simulink model "PV_Geno_VSC_GFL_634"  (R2024b)
settings: Solver=ode5  StartTime=0.0  StopTime=5  MaxStep=1e-4  RelTol=1e-6  AbsTol=1e-8
values from neighbouring files (symbols this model uses):
  a = 1.3    [init_para_with_symmtrc_loads.m]
  amp_ptb = amp_rel*Vp    [a01_scan_VSC_13_feeder.m]
  Cdc = 278e-3    (= 0.278)    [init_para_with_symmtrc_loads.m]
  fg = 60    [a01_scan_VSC_13_feeder.m]    (also in init_para_with_symmtrc_loads.m)
  Gn = 1000    [init_para_with_symmtrc_loads.m]
  Ipv_n = Isc_n*(Rp+Rs)/Rp    (= 8.21426513558)    [init_para_with_symmtrc_loads.m]
  Isc_n = 8.21    [init_para_with_symmtrc_loads.m]
  k = 1.3806503e-23    [init_para_with_symmtrc_loads.m]    (also in ypm_plot_compare_ana_meas.m = 2)
  KI = 0.0032    [init_para_with_symmtrc_loads.m]
  Ki_C = Rc/tau_C    (= 0.768)    [init_para_with_symmtrc_loads.m]
  Ki_DC = omega_DC^2*Cdc    [init_para_with_symmtrc_loads.m]
  Ki_P = 1/(Ki_pq*tau_P)    [init_para_with_symmtrc_loads.m]
  Ki_PLL = Kp_PLL/tau_PLL    [init_para_with_symmtrc_loads.m]
  Kp_C = Lc/tau_C    (= 0.020372)    [init_para_with_symmtrc_loads.m]
  Kp_DC = 2*xi_DC*omega_DC*Cdc    [init_para_with_symmtrc_loads.m]
  Kp_P = tau_C/(Ki_pq*tau_P)    [init_para_with_symmtrc_loads.m]
  Kp_PLL = xi_PLL*2*omega_PLL/Vp    [init_para_with_symmtrc_loads.m]
  KV = -0.123    [init_para_with_symmtrc_loads.m]
  KVmp = Vmp_n/Voc_n    (= 0.799392097264)    [init_para_with_symmtrc_loads.m]
  Lc = 20.372e-6    (= 2.0372e-05)    [init_para_with_symmtrc_loads.m]
  Np = 345    [init_para_with_symmtrc_loads.m]
  Ns = 45    [init_para_with_symmtrc_loads.m]
  Ns_cell = 54    [init_para_with_symmtrc_loads.m]
  phi_ptb = phi_ptb_vec(run)    [a01_scan_VSC_13_feeder.m]
  phs0 = mod(-w_ptb*t_start, 2*pi)    [a01_scan_VSC_13_feeder.m]
  psi_0 = 0    [a01_scan_VSC_13_feeder.m]
  q = 1.6021764e-19    [init_para_with_symmtrc_loads.m]
  Rc = 0.768e-3    (= 0.000768)    [init_para_with_symmtrc_loads.m]
  Rp = 425.405    [init_para_with_symmtrc_loads.m]
  Rs = 0.221    [init_para_with_symmtrc_loads.m]
  S_base_all = 1    [init_para_with_symmtrc_loads.m]
  t_start = t_settle    (= 0.5)    [a01_scan_VSC_13_feeder.m]
  Tn = 25    [init_para_with_symmtrc_loads.m]
  Ts = T_ctrl/n_ctrl    [a01_scan_VSC_13_feeder.m]    (also in init_para_with_symmtrc_loads.m = 5e-05)
  Vdc = 1200    [init_para_with_symmtrc_loads.m]
  Voc_n = 32.9    [init_para_with_symmtrc_loads.m]
  Vp = sqrt(2)*480/sqrt(3)    [a01_scan_VSC_13_feeder.m]    (also in init_para_with_symmtrc_loads.m = Ug*sqrt(2)/sqrt(3))
  w_ptb = 2*pi*fp    [a01_scan_VSC_13_feeder.m]
undefined symbols (not defined in the file or in its folder): Amp_ptb_A, Amp_ptb_B, Amp_ptb_C, DiscIntNeverNeededParam, frq_ptb_A, frq_ptb_B, frq_ptb_C, j, para_PVgeno, phs_ptb_A, phs_ptb_B, phs_ptb_C
libraries: spsControlledVoltageSourceLib x6, slpidlib x5, spsSeriesRLCBranchLib x4, spsPower3phInstantaneousLib x2, spsabctoAlphaBetaZeroLib x2, spsCurrentMeasurementLib x2, spsControlledCurrentSourceLib x2, spsGroundLib x1, spsVoltageMeasurementLib x1, spsThreePhaseVIMeasurementLib x1, spsThreePhaseParallelRLCLoadLib x1, spsThreePhaseSourceLib x1
(part 1 of 2)
settings Model: Creator=clubbert  LastModifiedBy=clubbert
settings DataIOCC: Decimation=D_log  SaveOutput=off  SaveState=on  DSMLogging=off

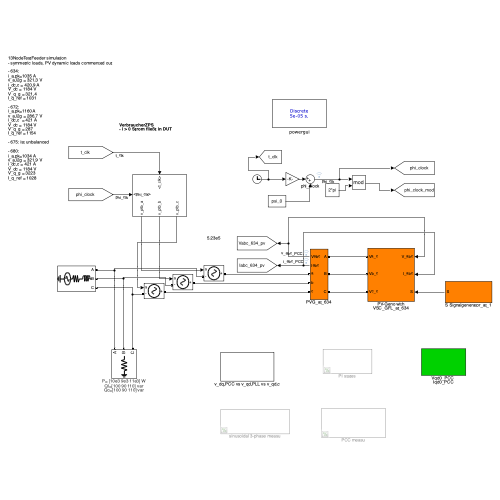
[thumbnail: Simulink's stored preview of the top-level diagram]
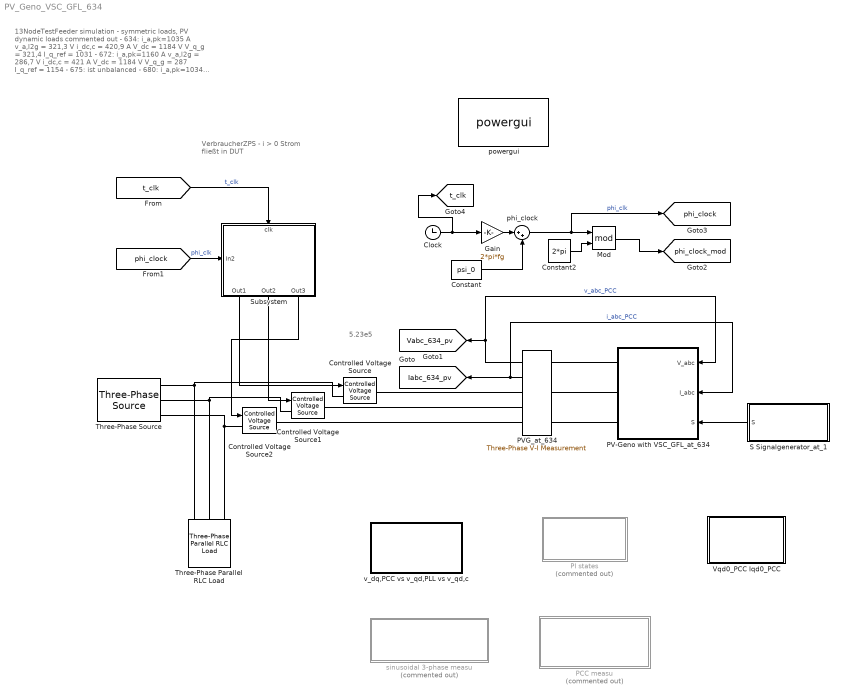
== system PV_Geno_VSC_GFL_634 ==
  note: VerbraucherZPS
      | - i > 0 Strom fließt in DUT
  note: 13NodeTestFeeder simulation
      | - symmetric loads, PV dynamic loads commented out
      |
      | - 634:
      | i_a,pk=1035 A
      | v_a,l2g = 321,3 V
      | i_dc,c = 420,9 A
      | V_dc = 1184 V
      | V_q_g = 321,4
      | I_q_ref = 1031
      |
      | - 672:
      | i_a,pk=1160 A
      | v_a,l2g = 286,7 V
      | i_dc,c  = 421 A
      | V_dc = 1184 V
      | V_q_g = 287
      | I_q_ref = 1154
      |
      | - 675: ist unbalanced
      |
      | - 680:
      | i_a,pk=1034 A
      | v_a,l2g = 321,9 V
      | i_dc,c = 421 A
      | V_dc = 1184 V
      | V_q_g = 3223
      | I_q_ref = 1028
  note: 5.23e5
  Clock : Clock
  Constant : Constant  Value=psi_0
  Constant2 : Constant  Value=2*pi
  Controlled Voltage Source : spsControlledVoltageSourceLib/Controlled Voltage Source  Initialize=on  Source_Type=AC  Amplitude=0  Phase=0  Frequency=0  Measurements=None
  Controlled Voltage Source1 : spsControlledVoltageSourceLib/Controlled Voltage Source  Initialize=on  Source_Type=AC  Amplitude=0  Phase=0  Frequency=0  Measurements=None
  Controlled Voltage Source2 : spsControlledVoltageSourceLib/Controlled Voltage Source  Initialize=on  Source_Type=AC  Amplitude=0  Phase=0  Frequency=0  Measurements=None
  Gain : Gain  Gain=2*pi*fg
  Mod : Math  Operator=mod
  PCC measu : Subsystem  Commented=on
  PI states : Subsystem  Commented=on
  "PV-Geno with VSC_GFL_at_634     " : Subsystem
      settings: PortSchema="{\"entries\":[{\"content\":{\"sides\":[{\"content\":{\"connectorIds\":[\"LConn1\",\"LConn2\",\"LConn3\"]},\"type\":\"ConnectorPlacement.EquallySpacedRectSide\",\"uuid\":\"92a05cf9-a19b-475d-bffb-9406018f82f4\"},{\"content\":{\"connectorIds\":[\"In1\",\"In2\",\"In3\"],\"side\":\"RIGHT\"},\"type\":\"ConnectorPlacement.EquallySpacedRectSide\",\"uuid\":\"83076eb6-0a86-49d7-8932-035501cdc6f6\"},{\"content\":{\"side\":\"TOP\"},\"type\":\"ConnectorPlacement.EquallySpacedRectSide\",\"uuid\":\"ba2310df-ee07-4a5c-88ff-ef0f81658322\"}]},\"type\":\"ConnectorPlacement.EquallySpacedConnector\",\"uuid\":\"9e64c472-0dae-4bb4-8eb3-3329c328d412\"}],\"packageUris\":[\"http://schema.mathworks.com/mf0/Connector/R2020b\"],\"version\":\"1.0\"}"
  PVG_at_634 : spsThreePhaseVIMeasurementLib/Three-Phase V-I Measurement  VoltageMeasurement=phase-to-ground  SetLabelV=off  LabelV=V_abc_PCC_634_pv  Vpu=off  VpuLL=off  CurrentMeasurement=yes  SetLabelI=off  LabelI=I_abc_PCC_634_pv  Ipu=off  Pbase=100e6  Vbase=4160  OutputType=Complex  PhasorSimulation=off  PSBequivalent=0
  S Signalgenerator_at_1 : Subsystem
  Subsystem : Subsystem
      settings: PortSchema="{\"entries\":[{\"content\":{\"sides\":[{\"content\":{\"connectorIds\":[\"In1\"]},\"type\":\"ConnectorPlacement.EquallySpacedRectSide\",\"uuid\":\"f4884b02-4acb-4d3a-a4cd-33952d0bc0e4\"},{\"content\":{\"connectorIds\":[\"Out1\",\"Out2\",\"Out3\"],\"side\":\"RIGHT\"},\"type\":\"ConnectorPlacement.EquallySpacedRectSide\",\"uuid\":\"6584eb96-7add-474a-938e-a48a378b8460\"},{\"content\":{\"connectorIds\":[\"In2\"],\"side\":\"TOP\"},\"type\":\"ConnectorPlacement.EquallySpacedRectSide\",\"uuid\":\"b17781d8-b149-4887-b17a-64ae556a6560\"}]},\"type\":\"ConnectorPlacement.EquallySpacedConnector\",\"uuid\":\"0fcb0f1f-785d-43c8-8af7-8220763653f1\"}],\"packageUris\":[\"http://schema.mathworks.com/mf0/Connector/R2020b\"],\"version\":\"1.0\"}"
  Three-Phase Parallel RLC Load : spsThreePhaseParallelRLCLoadLib/Three-Phase Parallel RLC Load  LConnTagsString=A|B|C  Configuration=Y (grounded)  NominalVoltage=480  Vabc=[1e3 1e3 1e3]  Vabcp=[1e3 1e3 1e3]  NominalFrequency=60  UnbalancedPower=off  ActivePower=4.969e+05  InductivePower=0  CapacitivePower=0  Pabc=[10e3 9e3 11e3]  QLabc=[100 90 110]  QCabc=[100 90 110]  Pabcp=[10e3 9e3 11e3]  QLabcp=[100 90 110]  QCabcp=[100 90 110]  Measurements=None  LoadType=constant Z
      settings: AttributesFormatString=|
      | P= %<Pabc> W
      | Ql=%<QLabc> var
      | Qc=%<QCabc> var
  Three-Phase Source : spsThreePhaseSourceLib/Three-Phase Source  InternalConnection=Yg  VoltagePhases=off  Voltage=480  PhaseAngle=0  Voltage_phases=[25e3 25e3 25e3]/sqrt(3)  PhaseAngles_phases=[0 -120 +120]  Frequency=60  NonIdealSource=on  SpecifyImpedance=on  Resistance=0.8929  Inductance=16.58e-3  ShortCircuitLevel=100e6  BaseVoltage=480  XRratio=7  BusType=swing  Pref=10e3  Qref=0  Prefabc=[10e3, 10e3, 10e3]  Qrefabc=[0, 0, 0]  Qmin=-inf  Qmax=inf
  Vqd0_PCC Iqd0_PCC : Subsystem
  phi_clock : Sum  Inputs=|++
  powergui : sps_lib/powergui  Priority=1  SimulationMode=Discrete  SampleTime=Ts  frequency=60  Iterations=50  frequencyindice=0  Pbase=100e3  ErrMax=0.0001  UnitsV=kV  UnitsW=kW  buscounter=0  FunctionMessages=off  echomessages=off  EnableUseOfTLC=off  CurrentSourceSwitches=off  DisableSnubberDevices=off  DisableRonSwitches=off  DisableVfSwitches=off  DisplayEquations=off  AutomaticDiscreteSolvers=off  SolverType=Tustin/Backward Euler (TBE)  Interpol=off  ExternalGateDelay=off  methode=off  Ts=0  x0status=blocks  SPID=off  SwTol=0  HookPort=off  NonlinearTolerance=1e-4  nMaxIteration=100  ContinueOnMaxIteration=off  RestoreLinks=warning  ResistiveCurrentMeasurement=off  Frange=[0:2:500]  Ylog=off  Xlog=on  ShowGrid=off  save=off  variable=ZData  structure=0  ZoomFFT=on  StartTime=0.0  cycles=1  DisplayStyle=1  fundamental=60  FreqAxis=off  MaxFrequency=1000  frequencyindicesteady=1  RmsSteady=1  display=off
  sinusoidal 3-phase measu : Subsystem  Commented=on
  v_dq,PCC vs v_qd,PLL vs v_qd,c : Subsystem
  tag scope: Iabc_634_pv=global, Vabc_634_pv=global, phi_clock=global, phi_clock_mod=global, t_clk=global
  wires:
  S Signalgenerator_at_1/1(S) -> "PV-Geno with VSC_GFL_at_634     "/3(S)
  PVG_at_634/1 -> "PV-Geno with VSC_GFL_at_634     "/1(V_abc), [Vabc_634_pv]  "v_abc_PCC"
  PVG_at_634/2 -> [Iabc_634_pv], "PV-Geno with VSC_GFL_at_634     "/2(I_abc)  "i_abc_PCC"
  Clock/1 -> [t_clk], Gain/1
  Gain/1 -> phi_clock/1
  phi_clock/1 -> Mod/1, [phi_clock]  "phi_clk"
  Constant/1 -> phi_clock/2
  Constant2/1 -> Mod/2
  Mod/1 -> [phi_clock_mod]
  Subsystem/1(Out1) -> Controlled Voltage Source/1
  Subsystem/2(Out2) -> Controlled Voltage Source1/1
  Subsystem/3(Out3) -> Controlled Voltage Source2/1
  [t_clk] -> Subsystem/1(clk)  "t_clk"
  [phi_clock] -> Subsystem/2(In2)  "phi_clk"
  connections:
  PVG_at_634/RConn3 -- Controlled Voltage Source2/RConn1
  "PV-Geno with VSC_GFL_at_634     "/LConn3 -- PVG_at_634/LConn3
  PVG_at_634/RConn2 -- Controlled Voltage Source1/RConn1
  PVG_at_634/RConn1 -- Controlled Voltage Source/RConn1
  "PV-Geno with VSC_GFL_at_634     "/LConn2 -- PVG_at_634/LConn2
  "PV-Geno with VSC_GFL_at_634     "/LConn1 -- PVG_at_634/LConn1
  Three-Phase Source/RConn1 -- Three-Phase Parallel RLC Load/LConn1 -- Controlled Voltage Source/LConn1
  Three-Phase Source/RConn2 -- Three-Phase Parallel RLC Load/LConn2 -- Controlled Voltage Source1/LConn1
  Three-Phase Source/RConn3 -- Three-Phase Parallel RLC Load/LConn3 -- Controlled Voltage Source2/LConn1

== system PV_Geno_VSC_GFL_634/PCC measu ==
  PQ_4 : Subsystem
  Scope1 : Scope
  Scope2 : Scope  NumInputPorts=2
  wires:
  PQ_4/1(PQ) -> Scope1/1  "PQ_at_634"
  [Iabc_634_pv] -> PQ_4/2(I), Scope2/2  "Iabc"
  [Vabc_634_pv] -> PQ_4/1(U), Scope2/1  "Vabc"

== system PV_Geno_VSC_GFL_634/PI states ==
  Constant : Constant  Value=2*pi*fg*0
  Scope3 : Scope  NumInputPorts=5
  Sum : Sum  Inputs=|++
  wires:
  [y_PI_PLL] -> Sum/2  "y_PI_PLL"
  [y_PI_q_CC] -> Scope3/4  "y_PI_q_CC"
  [y_PI_q_CC] -> Scope3/5  "y_PI_q_CC"
  [y_PI_DC] -> Scope3/2  "y_PI_DC"
  [y_PI_QC] -> Scope3/3  "y_PI_QC"
  Constant/1 -> Sum/1
  Sum/1 -> Scope3/1

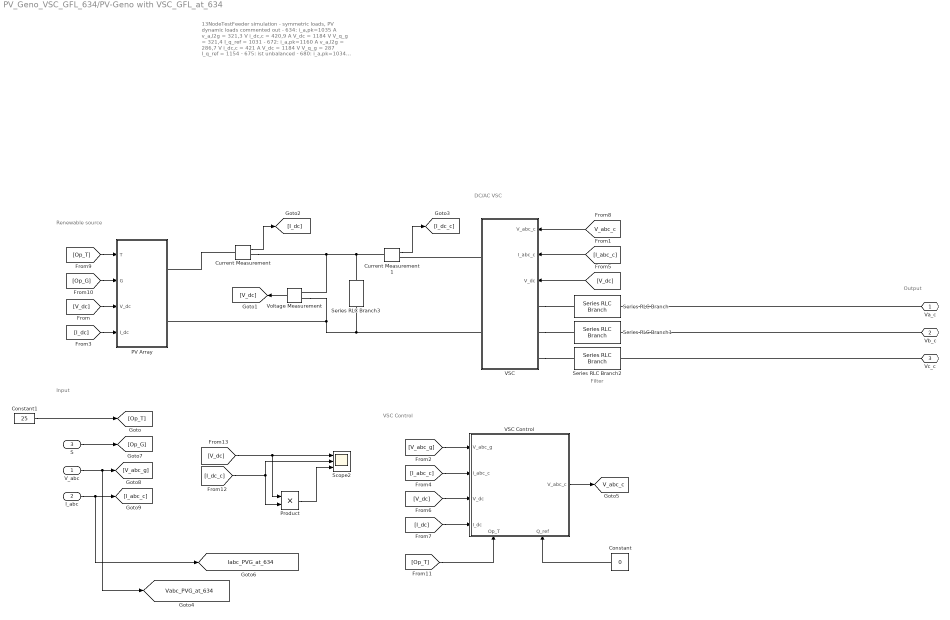
== system PV_Geno_VSC_GFL_634/PV-Geno with VSC_GFL_at_634      ==
  note: 13NodeTestFeeder simulation
      | - symmetric loads, PV dynamic loads commented out
      |
      | - 634:
      | i_a,pk=1035 A
      | v_a,l2g = 321,3 V
      | i_dc,c = 420,9 A
      | V_dc = 1184 V
      | V_q_g = 321,4
      | I_q_ref = 1031
      |
      | - 672:
      | i_a,pk=1160 A
      | v_a,l2g = 286,7 V
      | i_dc,c  = 421 A
      | V_dc = 1184 V
      | V_q_g = 287
      | I_q_ref = 1154
      |
      | - 675: ist unbalanced
      |
      | - 680:
      | i_a,pk=1034 A
      | v_a,l2g = 321,9 V
      | i_dc,c = 421 A
      | V_dc = 1184 V
      | V_q_g = 3223
      | I_q_ref = 1028
  note: Output
  note: Input
  note: Filter
  note: Renewable source
  note: VSC Control
  note: DC/AC VSC
  V_abc : Inport
  I_abc : Inport  Port=2
  S : Inport  Port=3
  Constant : Constant  Value=0
  Constant1 : Constant  Value=25
  Current Measurement : spsCurrentMeasurementLib/Current Measurement  PhasorSimulation=off  OutputType=Complex  PSBequivalent=0
  Current Measurement1 : spsCurrentMeasurementLib/Current Measurement  PhasorSimulation=off  OutputType=Complex  PSBequivalent=0
  PV Array : Subsystem
  Product : Product
  Scope2 : Scope  NumInputPorts=3
  Series RLC Branch : spsSeriesRLCBranchLib/Series RLC Branch  LConnTagsString=__new0  RConnTagsString=__new0  BranchType=RL  Resistance=Rc  Inductance=Lc  SetiL0=off  InitialCurrent=0  Capacitance=1e-6  Setx0=off  InitialVoltage=0  Measurements=None
  Series RLC Branch1 : spsSeriesRLCBranchLib/Series RLC Branch  LConnTagsString=__new0  RConnTagsString=__new0  BranchType=RL  Resistance=Rc  Inductance=Lc  SetiL0=off  InitialCurrent=0  Capacitance=1e-6  Setx0=off  InitialVoltage=0  Measurements=None
  Series RLC Branch2 : spsSeriesRLCBranchLib/Series RLC Branch  LConnTagsString=__new0  RConnTagsString=__new0  BranchType=RL  Resistance=Rc  Inductance=Lc  SetiL0=off  InitialCurrent=0  Capacitance=1e-6  Setx0=off  InitialVoltage=0  Measurements=None
  Series RLC Branch3 : spsSeriesRLCBranchLib/Series RLC Branch  LConnTagsString=__new0  RConnTagsString=__new0  BranchType=C  Resistance=0.3  Inductance=1e-3  SetiL0=off  InitialCurrent=0  Capacitance=Cdc  Setx0=on  InitialVoltage=Vdc  Measurements=None
  VSC : Subsystem
  VSC Control : Subsystem
      settings: PortSchema="{\"entries\":[{\"content\":{\"sides\":[{\"content\":{\"connectorIds\":[\"In1\",\"In2\",\"In3\",\"In4\"]},\"type\":\"ConnectorPlacement.EquallySpacedRectSide\",\"uuid\":\"1f0c866f-1355-4493-8a8b-fecd52da2e06\"},{\"content\":{\"connectorIds\":[\"Out1\"],\"side\":\"RIGHT\"},\"type\":\"ConnectorPlacement.EquallySpacedRectSide\",\"uuid\":\"e0482316-46fe-491c-835b-46d73fa6817a\"},{\"content\":{\"side\":\"TOP\"},\"type\":\"ConnectorPlacement.EquallySpacedRectSide\",\"uuid\":\"b85aba4d-c629-42a9-b30e-3179992b26cb\"},{\"content\":{\"connectorIds\":[\"In5\",\"In6\"],\"side\":\"BOTTOM\"},\"type\":\"ConnectorPlacement.EquallySpacedRectSide\",\"uuid\":\"2c79aeba-fb98-4b17-8331-d72a75796cf8\"}]},\"type\":\"ConnectorPlacement.EquallySpacedConnector\",\"uuid\":\"5586ce08-6872-4275-b1b0-323c6fc0897a\"}],\"packageUris\":[\"http://schema.mathworks.com/mf0/Connector/R2020b\"],\"version\":\"1.0\"}"
  Voltage Measurement : spsVoltageMeasurementLib/Voltage Measurement  PhasorSimulation=off  OutputType=Complex  PSBequivalent=0
  Va_c : PMIOPort  Side=Left
  Vb_c : PMIOPort  Port=2  Side=Left
  Vc_c : PMIOPort  Port=3  Side=Left
  tag scope: Iabc_PVG_at_634=global, V_abc_c=global, Vabc_PVG_at_634=global
  wires:
  [V_abc_c] -> VSC/1(V_abc_c)
  Constant/1 -> VSC Control/6(Q_ref)
  Current Measurement1/1 -> [I_dc_c]
  [V_dc] -> Scope2/1, Product/1
  [I_dc_c] -> Scope2/2, Product/2
  [I_dc] -> VSC Control/4(I_dc)
  Voltage Measurement/1 -> [V_dc]
  [V_abc_g] -> VSC Control/1(V_abc_g)
  VSC Control/1(V_abc_c) -> [V_abc_c]
  [V_dc] -> PV Array/3(V_dc)
  Current Measurement/1 -> [I_dc]
  Product/1 -> Scope2/3
  [Op_T] -> VSC Control/5(Op_T)
  [V_dc] -> VSC/3(V_dc)
  V_abc/1 -> [Vabc_PVG_at_634], [V_abc_g]
  [Op_T] -> PV Array/1(T)
  [V_dc] -> VSC Control/3(V_dc)
  [Op_G] -> PV Array/2(G)
  [I_abc_c] -> VSC Control/2(I_abc_c)
  [I_abc_c] -> VSC/2(I_abc_c)
  [I_dc] -> PV Array/4(I_dc)
  S/1 -> [Op_G]
  Constant1/1 -> [Op_T]
  I_abc/1 -> [Iabc_PVG_at_634], [I_abc_c]
  connections:
  VSC/LConn2 -- Series RLC Branch1/RConn1
  Series RLC Branch3/RConn1 -- Voltage Measurement/LConn2 -- PV Array/RConn2 -- VSC/RConn2
  Current Measurement1/LConn1 -- Series RLC Branch3/LConn1 -- Current Measurement/RConn1 -- Voltage Measurement/LConn1
  Current Measurement/LConn1 -- PV Array/RConn1
  VSC/LConn1 -- Series RLC Branch/RConn1
  VSC/LConn3 -- Series RLC Branch2/RConn1
  Va_c/RConn1 -- Series RLC Branch/LConn1
  VSC/RConn1 -- Current Measurement1/RConn1
  Vc_c/RConn1 -- Series RLC Branch2/LConn1
  Vb_c/RConn1 -- Series RLC Branch1/LConn1

== system PV_Geno_VSC_GFL_634/S Signalgenerator_at_1 ==
  Constant : Constant  Value=para_PVgeno.S_ini1
  Product : Product  Commented=on
  Signal Generator : SignalGenerator  Commented=on  Amplitude=50  Frequency=0.25
  Step : Step  Commented=on  Time=para_PVgeno.t_step  After=para_PVgeno.S_step  SampleTime=0
  Step1 : Step  Commented=on  Time=para_PVgeno.t_step11  After=para_PVgeno.S_step11  SampleTime=0
  Step2 : Step  Time=para_PVgeno.t_step12  After=para_PVgeno.S_step12  SampleTime=0
  Sum : Sum  Inputs=|++++
  S : Outport
  wires:
  Sum/1 -> S/1
  Constant/1 -> Sum/1
  Step2/1 -> Sum/3
  Step1/1 -> Product/1
  Signal Generator/1 -> Product/2
  Product/1 -> Sum/2
  Step/1 -> Sum/4

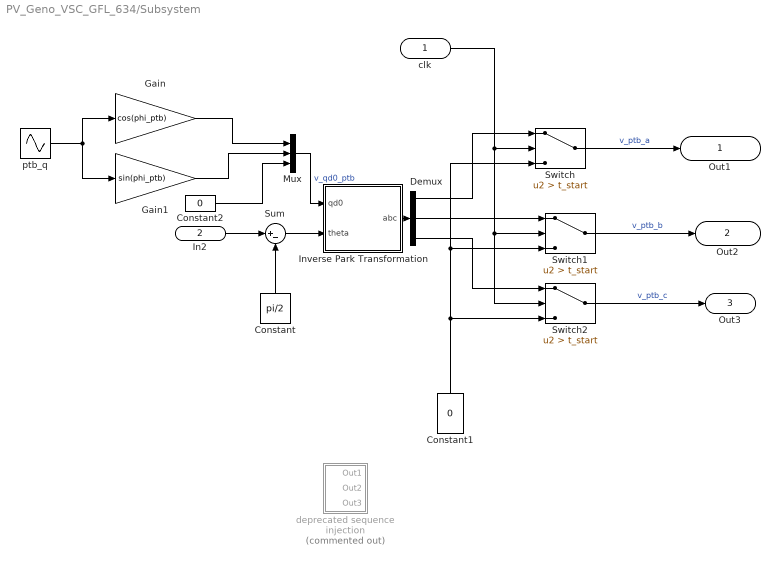
== system PV_Geno_VSC_GFL_634/Subsystem ==
  clk : Inport
  In2 : Inport  Port=2
  Constant : Constant  Value=pi/2
  Constant1 : Constant  Value=0
  Constant2 : Constant  Value=0
  Demux : Demux  Outputs=3
  Gain : Gain  Gain=cos(phi_ptb)
  Gain1 : Gain  Gain=sin(phi_ptb)
  Inverse Park Transformation : Subsystem
  Mux : Mux  Inputs=3
  Sum : Sum  Inputs=|+-
  Switch : Switch  Criteria=u2 > Threshold  Threshold=t_start  SaturateOnIntegerOverflow=off  InputSameDT=off
  Switch1 : Switch  Criteria=u2 > Threshold  Threshold=t_start  SaturateOnIntegerOverflow=off  InputSameDT=off
  Switch2 : Switch  Criteria=u2 > Threshold  Threshold=t_start  SaturateOnIntegerOverflow=off  InputSameDT=off
  deprecated sequence injection : Subsystem  Commented=on
  ptb_q : Sin  Amplitude=amp_ptb  Frequency=w_ptb  Phase=phs0  SampleTime=0
  Out1 : Outport
  Out2 : Outport  Port=2
  Out3 : Outport  Port=3
  wires:
  Switch1/1 -> Out2/1  "v_ptb_b"
  clk/1 -> Switch2/2, Switch1/2, Switch/2
  Switch/1 -> Out1/1  "v_ptb_a"
  Switch2/1 -> Out3/1  "v_ptb_c"
  Constant1/1 -> Switch2/3, Switch1/3, Switch/3
  Constant/1 -> Sum/2
  Sum/1 -> Inverse Park Transformation/2(theta)
  Inverse Park Transformation/1(abc) -> Demux/1
  Demux/1 -> Switch/1
  Demux/3 -> Switch2/1
  Demux/2 -> Switch1/1
  Constant2/1 -> Mux/3
  Mux/1 -> Inverse Park Transformation/1(qd0)  "v_qd0_ptb"
  In2/1 -> Sum/1
  ptb_q/1 -> Gain1/1, Gain/1
  Gain/1 -> Mux/1
  Gain1/1 -> Mux/2

== system PV_Geno_VSC_GFL_634/Vqd0_PCC Iqd0_PCC ==
  Constant1 : Constant  Value=pi/2
  Park Transformation I_PCC : Subsystem
      settings: PortSchema="{\"entries\":[{\"content\":{\"sides\":[{\"content\":{\"connectorIds\":[\"In1\"]},\"type\":\"ConnectorPlacement.EquallySpacedRectSide\",\"uuid\":\"413938a8-187c-4030-8e7b-ccf056000adc\"},{\"content\":{\"connectorIds\":[\"Out1\"],\"side\":\"RIGHT\"},\"type\":\"ConnectorPlacement.EquallySpacedRectSide\",\"uuid\":\"b1494641-b903-43ea-bd1f-2153ef0abf5c\"},{\"content\":{\"connectorIds\":[\"In2\"],\"side\":\"TOP\"},\"type\":\"ConnectorPlacement.EquallySpacedRectSide\",\"uuid\":\"8df33371-6fec-4d12-b754-42c64e56bccb\"}]},\"type\":\"ConnectorPlacement.EquallySpacedConnector\",\"uuid\":\"ccb4f1e5-dd19-4d52-8097-0d8dc2929079\"}],\"packageUris\":[\"http://schema.mathworks.com/mf0/Connector/R2020b\"],\"version\":\"1.0\"}"
  Park Transformation v_PCC : Subsystem
  Sum1 : Sum  Inputs=|+-
  tag scope: Iqd0_634_pv=global, Vqd0_634_pv=global
  wires:
  [Iabc_634_pv] -> Park Transformation I_PCC/1(abc)
  Constant1/1 -> Sum1/2
  [phi_clock] -> Sum1/1
  Park Transformation v_PCC/1(qd0) -> [Vqd0_634_pv]  "Vqd0_634_pv"
  Park Transformation I_PCC/1(qd0) -> [Iqd0_634_pv]  "Iqd0_634_pv"
  [Vabc_634_pv] -> Park Transformation v_PCC/1(abc)
  Sum1/1 -> Park Transformation I_PCC/2(theta), Park Transformation v_PCC/2(theta)

== system PV_Geno_VSC_GFL_634/sinusoidal 3-phase measu ==
  Constant2 : Constant  Value=2*pi
  Mod : Math  Operator=mod
  Mux : Mux  Inputs=2
  Scope : Scope  NumInputPorts=2
  Sum1 : Sum  Inputs=|+-
  wires:
  Constant2/1 -> Mod/2
  Mux/1 -> Scope/1  "phi phi_PLL pih_clk"
  [phi_clock] -> Sum1/2, Mux/2
  [theta_g] -> Mux/1, Sum1/1
  Sum1/1 -> Scope/2  "theta_PLL - phi_clk"

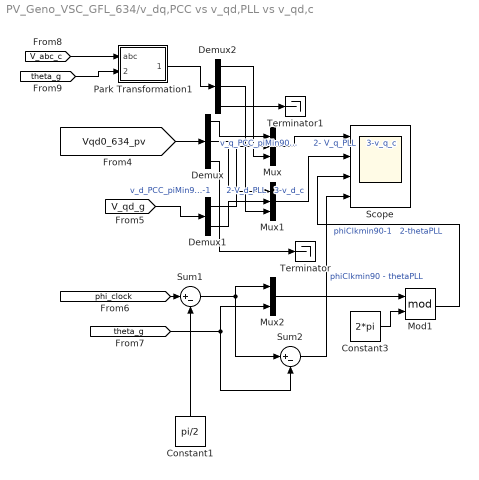
== system PV_Geno_VSC_GFL_634/v_dq,PCC vs v_qd,PLL vs v_qd,c ==
  Constant1 : Constant  Value=pi/2
  Constant3 : Constant  Value=2*pi
  Demux : Demux  Outputs=3
  Demux1 : Demux  Outputs=2
  Demux2 : Demux  Outputs=3
  Mod1 : Math  Operator=mod
  Mux : Mux  Inputs=3
  Mux1 : Mux  Inputs=3
  Mux2 : Mux  Inputs=2
  Park Transformation1 : Subsystem
  Scope : Scope  NumInputPorts=4
  Sum1 : Sum  Inputs=|+-
  Sum2 : Sum  Inputs=|+-
  Terminator : Terminator
  Terminator1 : Terminator
  wires:
  [Vqd0_634_pv] -> Demux/1
  Constant3/1 -> Mod1/2
  Demux2/3 -> Terminator1/1
  Demux1/1 -> Mux/2
  Demux1/2 -> Mux1/2
  Demux2/2 -> Mux1/3
  Sum2/1 -> Scope/4  "phiClkmin90 - thetaPLL"
  Mux/1 -> Scope/1  "v_q_PCC_piMin90-1      2- V_q_PLL    3-v_q_c"
  [theta_g] -> Park Transformation1/2(theta)
  Mux1/1 -> Scope/2  "v_d_PCC_piMin90-1      2-V_d_PLL   3-v_d_c"
  [V_abc_c] -> Park Transformation1/1(abc)
  Demux/2 -> Mux1/1
  Mod1/1 -> Scope/3  "phiClkmin90-1   2-thetaPLL"
  Demux/1 -> Mux/1
  [V_qd_g] -> Demux1/1
  [theta_g] -> Sum2/2, Mux2/2
  Mux2/1 -> Mod1/1
  Park Transformation1/1(qd0) -> Demux2/1
  Demux/3 -> Terminator/1
  Demux2/1 -> Mux/3
  [phi_clock] -> Sum1/1
  Sum1/1 -> Mux2/1, Sum2/1
  Constant1/1 -> Sum1/2

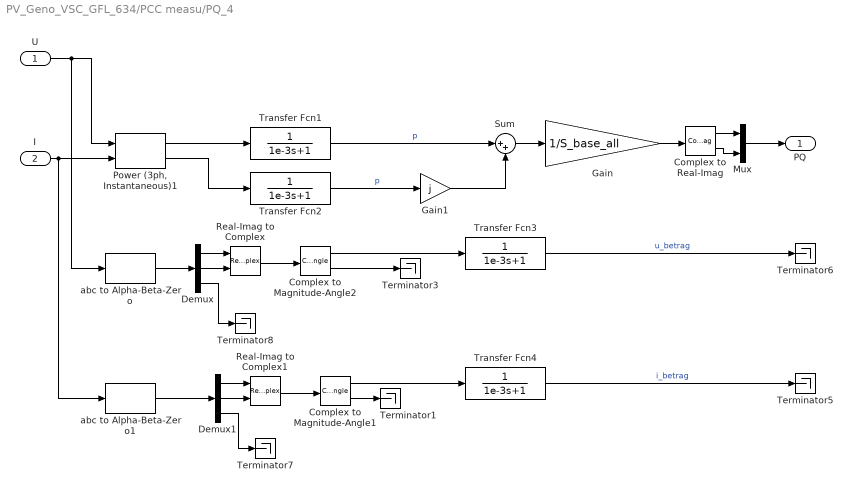
== system PV_Geno_VSC_GFL_634/PCC measu/PQ_4 ==
  U : Inport
  I : Inport  Port=2
  Complex to Magnitude-Angle1 : ComplexToMagnitudeAngle
  Complex to Magnitude-Angle2 : ComplexToMagnitudeAngle
  Complex to Real-Imag : ComplexToRealImag
  Demux : Demux  Outputs=3
  Demux1 : Demux  Outputs=3
  Gain : Gain  Gain=1/S_base_all
  Gain1 : Gain  Gain=j
  Mux : Mux  Inputs=2
  "Power (3ph, Instantaneous)1" : spsPower3phInstantaneousLib/Power (3ph, Instantaneous)
  Real-Imag to Complex : RealImagToComplex
  Real-Imag to Complex1 : RealImagToComplex
  Sum : Sum  Inputs=|++
  Terminator{1,3,5..8} (6 alike) : Terminator
  Transfer Fcn{1..4} (4 alike) : TransferFcn  Denominator=[1e-3 1]
  abc to Alpha-Beta-Zero : spsabctoAlphaBetaZeroLib/abc to Alpha-Beta-Zero
  abc to Alpha-Beta-Zero1 : spsabctoAlphaBetaZeroLib/abc to Alpha-Beta-Zero
  PQ : Outport
  wires:
  I/1 -> abc to Alpha-Beta-Zero1/1, "Power (3ph, Instantaneous)1"/2
  Gain1/1 -> Sum/2
  Complex to Real-Imag/1 -> Mux/1
  Complex to Real-Imag/2 -> Mux/2
  Mux/1 -> PQ/1
  "Power (3ph, Instantaneous)1"/2 -> Transfer Fcn2/1
  "Power (3ph, Instantaneous)1"/1 -> Transfer Fcn1/1
  Sum/1 -> Gain/1
  Gain/1 -> Complex to Real-Imag/1
  U/1 -> abc to Alpha-Beta-Zero/1, "Power (3ph, Instantaneous)1"/1
  abc to Alpha-Beta-Zero/1 -> Demux/1
  Demux/1 -> Real-Imag to Complex/1
  Demux/2 -> Real-Imag to Complex/2
  Real-Imag to Complex/1 -> Complex to Magnitude-Angle2/1
  Complex to Magnitude-Angle2/1 -> Transfer Fcn3/1
  Complex to Magnitude-Angle2/2 -> Terminator3/1
  Complex to Magnitude-Angle1/1 -> Transfer Fcn4/1
  Real-Imag to Complex1/1 -> Complex to Magnitude-Angle1/1
  Demux1/2 -> Real-Imag to Complex1/2
  Demux1/1 -> Real-Imag to Complex1/1
  abc to Alpha-Beta-Zero1/1 -> Demux1/1
  Transfer Fcn1/1 -> Sum/1  "p"
  Transfer Fcn2/1 -> Gain1/1  "p"
  Transfer Fcn3/1 -> Terminator6/1  "u_betrag"
  Transfer Fcn4/1 -> Terminator5/1  "i_betrag"
  Demux1/3 -> Terminator7/1
  Demux/3 -> Terminator8/1
  Complex to Magnitude-Angle1/2 -> Terminator1/1

== system PV_Geno_VSC_GFL_634/PV-Geno with VSC_GFL_at_634     /PV Array ==
  note: Allows PV model to initialize
  T : Inport
  G : Inport  Port=2
  V_dc : Inport  Port=3
  I_dc : Inport  Port=4
  Controlled Current Source19 : spsControlledCurrentSourceLib/Controlled Current Source  Initialize=on  Source_Type=AC  Amplitude=0  Phase=0  Frequency=0  Measurements=None
  Display : Display
  I module : MATLABFcn  MATLABFcn=Np*u(2)-Np*u(1)*(exp((u(3)/(Ns)+Rs*u(4)/Np)/((Ns_cell*k*(u(5)+273.15)/q)*a))-1)-Np*((u(3)/(Ns)+Rs*u(4)/Np)/Rp)  OutputDimensions=1
  I0 : MATLABFcn  MATLABFcn=(Isc_n+KI*(u(1)-Tn))/(exp((Voc_n+KV*(u(1)-Tn))/((Ns_cell*k*(u(1)+273.15)/q)*a))-1);  OutputDimensions=1
  Ipv : MATLABFcn  MATLABFcn=(Ipv_n+KI*(u(1)-Tn))*(u(2)/Gn);  OutputDimensions=1
  Memory : Memory
  Memory1 : Memory
  Mux : Mux  Inputs=2
  Mux1 : Mux  Inputs=5
  Product17 : Product
  Saturation : Saturate  UpperLimit=10e6  LowerLimit=0.1
  Step16 : Step  Time=0.001  SampleTime=0
  PV+ : PMIOPort  Side=Right
  PV- : PMIOPort  Port=2  Side=Right
  wires:
  Mux1/1 -> I module/1
  G/1 -> Mux/2
  Mux/1 -> Ipv/1
  T/1 -> Mux1/5, Mux/1, I0/1
  Ipv/1 -> Mux1/2
  I0/1 -> Mux1/1
  Memory/1 -> Mux1/4
  I_dc/1 -> Memory/1
  Saturation/1 -> Product17/1
  Step16/1 -> Product17/2
  Product17/1 -> Controlled Current Source19/1
  Memory1/1 -> Mux1/3
  V_dc/1 -> Memory1/1
  I module/1 -> Display/1, Saturation/1
  connections:
  PV+/RConn1 -- Controlled Current Source19/RConn1
  Controlled Current Source19/LConn1 -- PV-/RConn1

== system PV_Geno_VSC_GFL_634/PV-Geno with VSC_GFL_at_634     /VSC ==
  V_abc_c : Inport
  I_abc_c : Inport  Port=2
  V_dc : Inport  Port=3
  Controlled Current Source1 : spsControlledCurrentSourceLib/Controlled Current Source  Initialize=on  Source_Type=AC  Amplitude=0  Phase=0  Frequency=0  Measurements=None
  Controlled Voltage Source3 : spsControlledVoltageSourceLib/Controlled Voltage Source  Initialize=off  Source_Type=AC  Amplitude=0  Phase=0  Frequency=60  Measurements=None
  Controlled Voltage Source4 : spsControlledVoltageSourceLib/Controlled Voltage Source  Initialize=off  Source_Type=AC  Amplitude=0  Phase=0  Frequency=60  Measurements=None
  Controlled Voltage Source5 : spsControlledVoltageSourceLib/Controlled Voltage Source  Initialize=off  Source_Type=AC  Amplitude=0  Phase=0  Frequency=60  Measurements=None
  Delay : Delay  DelayLength=1  InitialCondition=1200
  Demux : Demux  Outputs=3
  Divide : Product  Inputs=*/  RndMeth=Zero  SaturateOnIntegerOverflow=on
  Ground : spsGroundLib/Ground  LConnTagsString=a
  Product : Product
  Sum of Elements : Sum  Inputs=+
  Va_c : PMIOPort  Side=Left
  Vb_c : PMIOPort  Port=2  Side=Left
  Vc_c : PMIOPort  Port=3  Side=Left
  dc+ : PMIOPort  Port=4  Side=Right
  dc- : PMIOPort  Port=5  Side=Right
  wires:
  Product/1 -> Sum of Elements/1
  I_abc_c/1 -> Product/2
  V_abc_c/1 -> Demux/1, Product/1
  Demux/2 -> Controlled Voltage Source4/1
  Demux/1 -> Controlled Voltage Source3/1
  Demux/3 -> Controlled Voltage Source5/1
  Sum of Elements/1 -> Divide/1
  Divide/1 -> Controlled Current Source1/1
  V_dc/1 -> Delay/1
  Delay/1 -> Divide/2
  connections:
  Vb_c/RConn1 -- Controlled Voltage Source4/RConn1
  Va_c/RConn1 -- Controlled Voltage Source3/RConn1
  Controlled Voltage Source4/LConn1 -- Controlled Voltage Source3/LConn1 -- Controlled Voltage Source5/LConn1 -- Ground/LConn1
  Vc_c/RConn1 -- Controlled Voltage Source5/RConn1
  Controlled Current Source1/RConn1 -- dc-/RConn1
  dc+/RConn1 -- Controlled Current Source1/LConn1

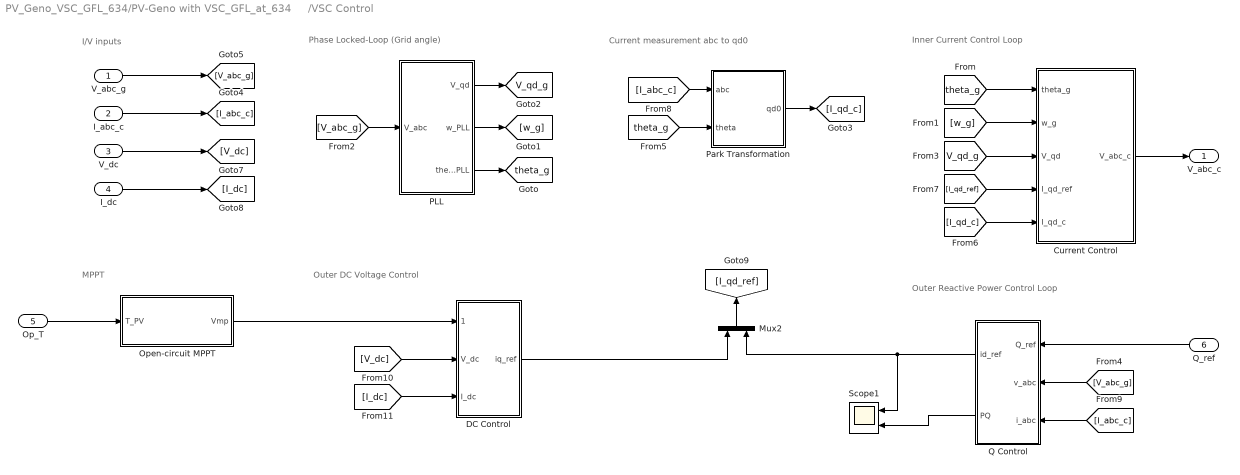
== system PV_Geno_VSC_GFL_634/PV-Geno with VSC_GFL_at_634     /VSC Control ==
  note: I/V inputs
  note: Phase Locked-Loop (Grid angle)
  note: Current measurement abc to qd0
  note: Inner Current Control Loop
  note: Outer Reactive Power Control Loop
  note: MPPT
  note: Outer DC Voltage Control
  V_abc_g : Inport
  I_abc_c : Inport  Port=2
  V_dc : Inport  Port=3
  I_dc : Inport  Port=4
  Op_T : Inport  Port=5
  Q_ref : Inport  Port=6
  Current Control : Subsystem
  DC Control : Subsystem
  Mux2 : Mux  Inputs=2
  Open-circuit MPPT : Subsystem
  PLL : Subsystem
  Park Transformation : Subsystem
  Q Control : Subsystem
  Scope1 : Scope  NumInputPorts=2
  V_abc_c : Outport
  tag scope: V_qd_g=global, theta_g=global
  wires:
  Park Transformation/1(qd0) -> [I_qd_c]
  [theta_g] -> Current Control/1(theta_g)
  PLL/3(theta_PLL) -> [theta_g]
  [I_qd_ref] -> Current Control/4(I_qd_ref)
  [theta_g] -> Park Transformation/2(theta)
  PLL/1(V_qd) -> [V_qd_g]
  PLL/2(w_PLL) -> [w_g]
  [w_g] -> Current Control/2(w_g)
  [V_qd_g] -> Current Control/3(V_qd)
  [I_qd_c] -> Current Control/5(I_qd_c)
  Current Control/1(V_abc_c) -> V_abc_c/1
  [V_abc_g] -> Q Control/2(v_abc)
  [I_abc_c] -> Q Control/3(i_abc)
  [V_dc] -> DC Control/2(V_dc)
  [I_dc] -> DC Control/3(I_dc)
  [I_abc_c] -> Park Transformation/1(abc)
  V_dc/1 -> [V_dc]
  I_abc_c/1 -> [I_abc_c]
  V_abc_g/1 -> [V_abc_g]
  I_dc/1 -> [I_dc]
  DC Control/1(iq_ref) -> Mux2/1
  Mux2/1 -> [I_qd_ref]
  Q_ref/1 -> Q Control/1(Q_ref)
  Op_T/1 -> Open-circuit MPPT/1(T_PV)
  Q Control/2(PQ) -> Scope1/2
  Open-circuit MPPT/1(Vmp) -> DC Control/1(V_dc_ref)
  [V_abc_g] -> PLL/1(V_abc)
  Q Control/1(id_ref) -> Scope1/1, Mux2/2

== system PV_Geno_VSC_GFL_634/Subsystem/Inverse Park Transformation ==
  qd0 : Inport
  theta : Inport  Port=2
  Constant2 : Constant
  Constant3 : Constant  Value=2*pi/3
  Cos : Trigonometry  Operator=cos
  Matrix Concatenate : Concatenate  NumInputs=3  Mode=Multidimensional array  ConcatenateDimension=2
  Matrix Multiply : Product  Multiplication=Matrix(*)
  Mux1 : Mux  Inputs=3
  Mux2 : Mux  Inputs=3
  Sin : Trigonometry
  Sum : Sum  Inputs=+-|
  Sum1 : Sum  Inputs=++|
  abc : Outport
  wires:
  Constant3/1 -> Sum/2, Sum1/2
  theta/1 -> Mux1/1, Sum1/1, Sum/1
  qd0/1 -> Matrix Multiply/2
  Sum/1 -> Mux1/2
  Sum1/1 -> Mux1/3
  Matrix Multiply/1 -> abc/1
  Mux2/1 -> Matrix Concatenate/3
  Matrix Concatenate/1 -> Matrix Multiply/1
  Mux1/1 -> Cos/1, Sin/1
  Cos/1 -> Matrix Concatenate/1
  Constant2/1 -> Mux2/2, Mux2/3, Mux2/1
  Sin/1 -> Matrix Concatenate/2

== system PV_Geno_VSC_GFL_634/Subsystem/deprecated sequence injection ==
  ptb_A : Sin  Amplitude=Amp_ptb_A  Frequency=frq_ptb_A  Phase=phs_ptb_A  SampleTime=0
  ptb_B : Sin  Amplitude=Amp_ptb_B  Frequency=frq_ptb_B  Phase=phs_ptb_B  SampleTime=0
  ptb_C : Sin  Amplitude=Amp_ptb_C  Frequency=frq_ptb_C  Phase=phs_ptb_C  SampleTime=0
  Out1 : Outport
  Out2 : Outport  Port=2
  Out3 : Outport  Port=3
  wires:
  ptb_C/1 -> Out3/1
  ptb_A/1 -> Out1/1
  ptb_B/1 -> Out2/1

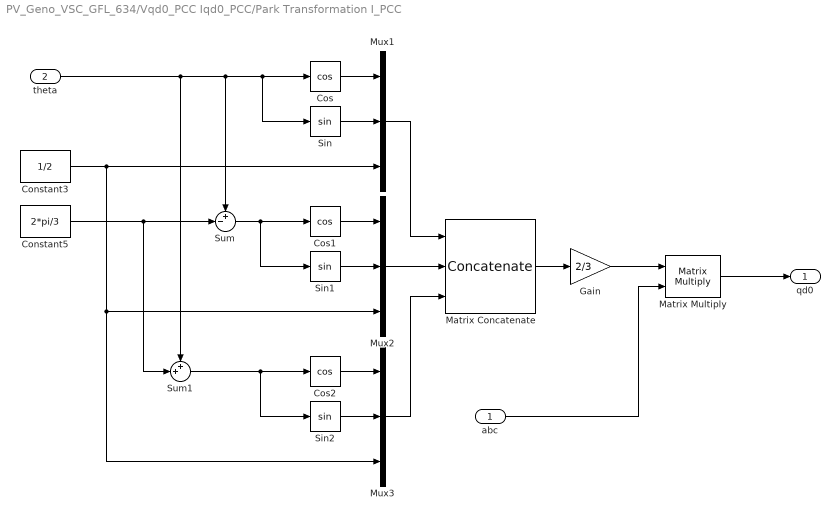
== system PV_Geno_VSC_GFL_634/Vqd0_PCC Iqd0_PCC/Park Transformation I_PCC ==
  abc : Inport
  theta : Inport  Port=2
  Constant3 : Constant  Value=1/2
  Constant5 : Constant  Value=2*pi/3
  Cos : Trigonometry  Operator=cos
  Cos1 : Trigonometry  Operator=cos
  Cos2 : Trigonometry  Operator=cos
  Gain : Gain  Gain=2/3
  Matrix Concatenate : Concatenate  NumInputs=3  Mode=Multidimensional array  ConcatenateDimension=2
  Matrix Multiply : Product  Multiplication=Matrix(*)
  Mux1 : Mux  Inputs=3
  Mux2 : Mux  Inputs=3
  Mux3 : Mux  Inputs=3
  Sin : Trigonometry
  Sin1 : Trigonometry
  Sin2 : Trigonometry
  Sum : Sum  Inputs=+-|
  Sum1 : Sum  Inputs=++|
  qd0 : Outport
  wires:
  Constant5/1 -> Sum1/2, Sum/2
  Matrix Multiply/1 -> qd0/1
  Matrix Concatenate/1 -> Gain/1
  Sin1/1 -> Mux2/2
  Mux3/1 -> Matrix Concatenate/3
  Cos1/1 -> Mux2/1
  Mux1/1 -> Matrix Concatenate/1
  Cos2/1 -> Mux3/1
  Sum/1 -> Cos1/1, Sin1/1
  Mux2/1 -> Matrix Concatenate/2
  Sin/1 -> Mux1/2
  Sin2/1 -> Mux3/2
  Constant3/1 -> Mux1/3, Mux2/3, Mux3/3
  theta/1 -> Sin/1, Cos/1, Sum/1, Sum1/1
  Gain/1 -> Matrix Multiply/1
  Cos/1 -> Mux1/1
  abc/1 -> Matrix Multiply/2
  Sum1/1 -> Cos2/1, Sin2/1

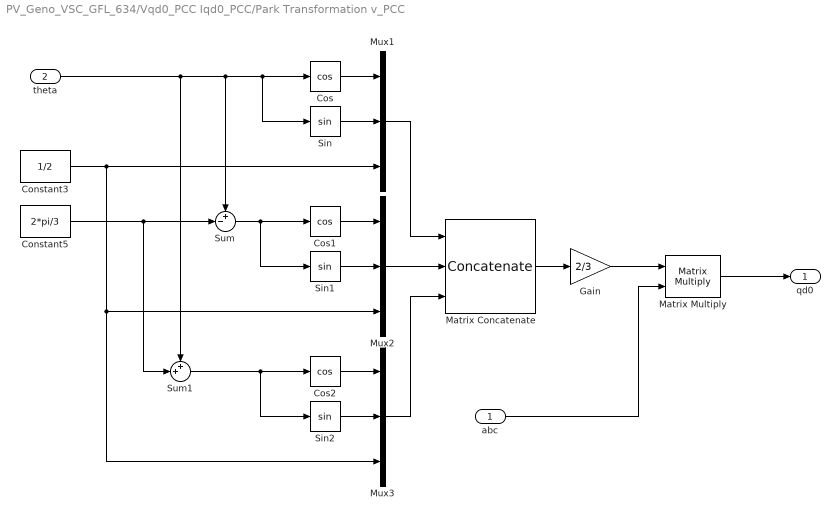
== system PV_Geno_VSC_GFL_634/Vqd0_PCC Iqd0_PCC/Park Transformation v_PCC ==
  abc : Inport
  theta : Inport  Port=2
  Constant3 : Constant  Value=1/2
  Constant5 : Constant  Value=2*pi/3
  Cos : Trigonometry  Operator=cos
  Cos1 : Trigonometry  Operator=cos
  Cos2 : Trigonometry  Operator=cos
  Gain : Gain  Gain=2/3
  Matrix Concatenate : Concatenate  NumInputs=3  Mode=Multidimensional array  ConcatenateDimension=2
  Matrix Multiply : Product  Multiplication=Matrix(*)
  Mux1 : Mux  Inputs=3
  Mux2 : Mux  Inputs=3
  Mux3 : Mux  Inputs=3
  Sin : Trigonometry
  Sin1 : Trigonometry
  Sin2 : Trigonometry
  Sum : Sum  Inputs=+-|
  Sum1 : Sum  Inputs=++|
  qd0 : Outport
  wires:
  Constant5/1 -> Sum1/2, Sum/2
  Matrix Multiply/1 -> qd0/1
  Matrix Concatenate/1 -> Gain/1
  Sin1/1 -> Mux2/2
  Mux3/1 -> Matrix Concatenate/3
  Cos1/1 -> Mux2/1
  Mux1/1 -> Matrix Concatenate/1
  Cos2/1 -> Mux3/1
  Sum/1 -> Cos1/1, Sin1/1
  Mux2/1 -> Matrix Concatenate/2
  Sin/1 -> Mux1/2
  Sin2/1 -> Mux3/2
  Constant3/1 -> Mux1/3, Mux2/3, Mux3/3
  theta/1 -> Sin/1, Cos/1, Sum/1, Sum1/1
  Gain/1 -> Matrix Multiply/1
  Cos/1 -> Mux1/1
  abc/1 -> Matrix Multiply/2
  Sum1/1 -> Cos2/1, Sin2/1

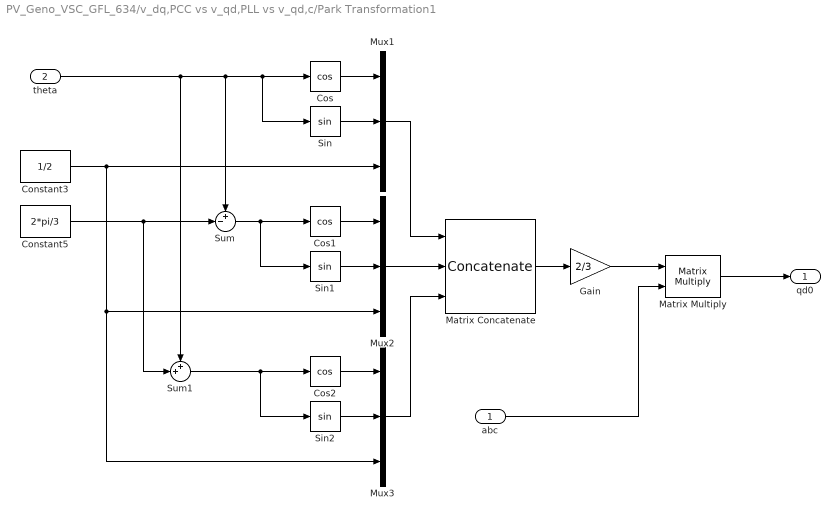
== system PV_Geno_VSC_GFL_634/v_dq,PCC vs v_qd,PLL vs v_qd,c/Park Transformation1 ==
  abc : Inport
  theta : Inport  Port=2
  Constant3 : Constant  Value=1/2
  Constant5 : Constant  Value=2*pi/3
  Cos : Trigonometry  Operator=cos
  Cos1 : Trigonometry  Operator=cos
  Cos2 : Trigonometry  Operator=cos
  Gain : Gain  Gain=2/3
  Matrix Concatenate : Concatenate  NumInputs=3  Mode=Multidimensional array  ConcatenateDimension=2
  Matrix Multiply : Product  Multiplication=Matrix(*)
  Mux1 : Mux  Inputs=3
  Mux2 : Mux  Inputs=3
  Mux3 : Mux  Inputs=3
  Sin : Trigonometry
  Sin1 : Trigonometry
  Sin2 : Trigonometry
  Sum : Sum  Inputs=+-|
  Sum1 : Sum  Inputs=++|
  qd0 : Outport
  wires:
  Constant5/1 -> Sum1/2, Sum/2
  Matrix Multiply/1 -> qd0/1
  Matrix Concatenate/1 -> Gain/1
  Sin1/1 -> Mux2/2
  Mux3/1 -> Matrix Concatenate/3
  Cos1/1 -> Mux2/1
  Mux1/1 -> Matrix Concatenate/1
  Cos2/1 -> Mux3/1
  Sum/1 -> Cos1/1, Sin1/1
  Mux2/1 -> Matrix Concatenate/2
  Sin/1 -> Mux1/2
  Sin2/1 -> Mux3/2
  Constant3/1 -> Mux1/3, Mux2/3, Mux3/3
  theta/1 -> Sin/1, Cos/1, Sum/1, Sum1/1
  Gain/1 -> Matrix Multiply/1
  Cos/1 -> Mux1/1
  abc/1 -> Matrix Multiply/2
  Sum1/1 -> Cos2/1, Sin2/1

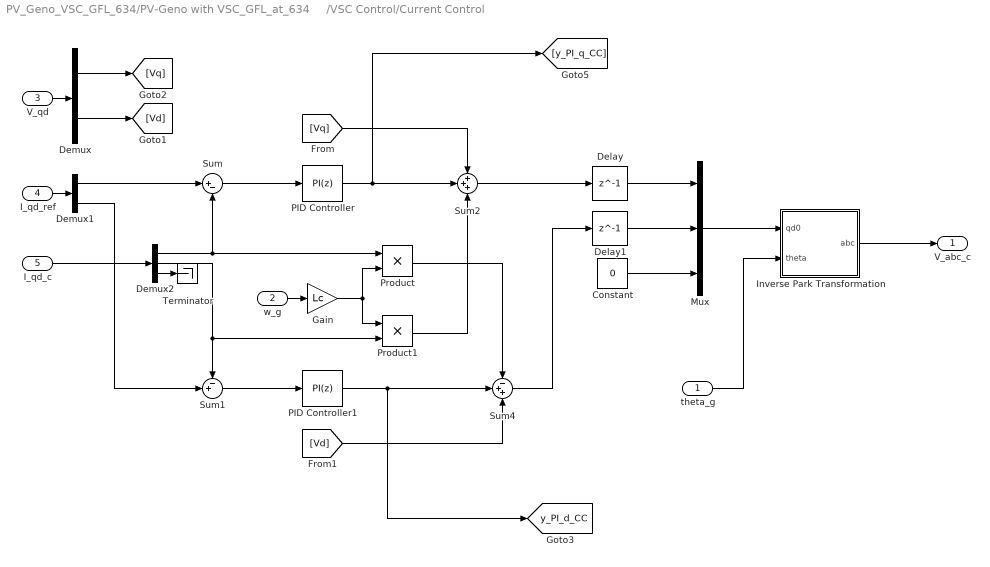
== system PV_Geno_VSC_GFL_634/PV-Geno with VSC_GFL_at_634     /VSC Control/Current Control ==
  theta_g : Inport
  w_g : Inport  Port=2
  V_qd : Inport  Port=3
  I_qd_ref : Inport  Port=4
  I_qd_c : Inport  Port=5
  Constant : Constant  Value=0
  Delay : Delay  DelayLength=1  InitialCondition=0.1
  Delay1 : Delay  DelayLength=1  InitialCondition=0.1
  Demux : Demux  Outputs=2
  Demux1 : Demux  Outputs=2
  Demux2 : Demux  Outputs=3
  Gain : Gain  Gain=Lc
  Inverse Park Transformation : Subsystem
  Mux : Mux  Inputs=3
  PID Controller : slpidlib/PID Controller  Controller=PI  Form=Parallel  TimeDomain=Discrete-time  UseExternalTs=off  SampleTime=Ts  IntegratorMethod=Forward Euler  FilterMethod=Forward Euler  ControllerParametersSource=internal  P=Kp_C  I=Ki_C  UseKiTs=off  D=0  UseExternalDerivativeSource=off  N=100  UseFilter=on  TunerSelectOption=Transfer Function Based (PID Tuner App)  InitialConditionSource=internal  InitialConditionForIntegrator=0  InitialConditionForFilter=0  DifferentiatorICPrevScaledInput=0  ExternalReset=none  TrackingMode=off  Kt=1  LimitOutput=off  SatLimitsSource=internal  UpperSaturationLimit=inf  LowerSaturationLimit=-inf  LinearizeAsGain=on  AntiWindupMode=none  Kb=1  LimitIntegrator=off  UpperIntegratorSaturationLimit=inf  LowerIntegratorSaturationLimit=-inf  POutMin=[]  POutMax=[]  IOutMin=[]  IOutMax=[]  DOutMin=[]  DOutMax=[]  NOutMin=[]  NOutMax=[]  SumOutMin=[]  SumOutMax=[]  SaturationOutMin=[]  SaturationOutMax=[]  PParamMin=[]  PParamMax=[]  IParamMin=[]  IParamMax=[]  DParamMin=[]  DParamMax=[]  NParamMin=[]  NParamMax=[]  KbParamMin=[]  KbParamMax=[]  KtParamMin=[]  KtParamMax=[]  KbOutMin=[]  KbOutMax=[]  KtOutMin=[]  KtOutMax=[]  IntegratorOutMin=[]  IntegratorOutMax=[]  FilterOutMin=[]  FilterOutMax=[]  SumI1OutMin=[]  SumI1OutMax=[]  SumI2OutMin=[]  SumI2OutMax=[]  SumI3OutMin=[]  SumI3OutMax=[]  SumI4OutMin=[]  SumI4OutMax=[]  SumDOutMin=[]  SumDOutMax=[]  DifferentiatorOutMin=[]  DifferentiatorOutMax=[]  FilterDiffOutCoefMin=[]  FilterDiffOutCoefMax=[]  ReciprocalOutMin=[]  ReciprocalOutMax=[]  SumDenOutMin=[]  SumDenOutMax=[]  SumNumOutMin=[]  SumNumOutMax=[]  DivideOutMin=[]  DivideOutMax=[]  UdiffTsProdOutMin=[]  UdiffTsProdOutMax=[]  NTsProdOutMin=[]  NTsProdOutMax=[]  UintegralTsProdOutMin=[]  UintegralTsProdOutMax=[]  UngainTsProdOutMin=[]  UngainTsProdOutMax=[]  ClampingZeroOutDataTypeStr=Inherit: Inherit via back propagation  ClampingZeroOutMin=[]  ClampingZeroOutMax=[]  FilterDenConstantOutDataTypeStr=Inherit: Inherit via back propagation  FilterDenConstantOutMin=[]  FilterDenConstantOutMax=[]  PCopyOutDataTypeStr=Inherit: Inherit via back propagation  PCopyOutMin=[]  PCopyOutMax=[]  NCopyOutDataTypeStr=Inherit: Inherit via back propagation  NCopyOutMin=[]  NCopyOutMax=[]  IntegratorContinuousStateAttributes=''  IntegratorStateMustResolveToSignalObject=off  IntegratorRTWStateStorageClass=Auto  FilterContinuousStateAttributes=''  FilterStateMustResolveToSignalObject=off  FilterRTWStateStorageClass=Auto  ParallelPVariant=InternalParameters  IdealPVariant=Disabled  IVariant=InternalParameters  DVariant=Disabled  IntegratorVariant=Discrete  SatVariant=Disabled  AWVariant=Passthrough  PCopyVariant=Disabled  TRVariant=Disabled  FdbkBlocksVariant=Forward  IdealPFdbkVariant=Disabled  SatFdbkVariant=Disabled  DerivativeFilterVariant=Disabled  NVariant=Disabled  NCopyVariant=Disabled_SignalSpec  FilterICVariant=Disabled  IntegratorICVariant=InternalICs  ExternalResetVariant=Disabled  TRSumVariant=Passthrough  SumFdbkVariant=Disabled  SumVariant=Sum_PI  TsampFilterVariant=InternalTs  TsampNgainVariant=Passthrough  TsampIntegralVariant=Disabled_SignalSpec  ExternalSaturationOutDataTypeStr=Inherit: Same as second input  DerivativeSourceVariant=Disabled  PreIntVariant=InternalPreInt
  PID Controller1 : slpidlib/PID Controller  Controller=PI  Form=Parallel  TimeDomain=Discrete-time  UseExternalTs=off  SampleTime=Ts  IntegratorMethod=Forward Euler  FilterMethod=Forward Euler  ControllerParametersSource=internal  P=Kp_C  I=Ki_C  UseKiTs=off  D=0  UseExternalDerivativeSource=off  N=100  UseFilter=on  TunerSelectOption=Transfer Function Based (PID Tuner App)  InitialConditionSource=internal  InitialConditionForIntegrator=0  InitialConditionForFilter=0  DifferentiatorICPrevScaledInput=0  ExternalReset=none  TrackingMode=off  Kt=1  LimitOutput=off  SatLimitsSource=internal  UpperSaturationLimit=inf  LowerSaturationLimit=-inf  LinearizeAsGain=on  AntiWindupMode=none  Kb=1  LimitIntegrator=off  UpperIntegratorSaturationLimit=inf  LowerIntegratorSaturationLimit=-inf  POutMin=[]  POutMax=[]  IOutMin=[]  IOutMax=[]  DOutMin=[]  DOutMax=[]  NOutMin=[]  NOutMax=[]  SumOutMin=[]  SumOutMax=[]  SaturationOutMin=[]  SaturationOutMax=[]  PParamMin=[]  PParamMax=[]  IParamMin=[]  IParamMax=[]  DParamMin=[]  DParamMax=[]  NParamMin=[]  NParamMax=[]  KbParamMin=[]  KbParamMax=[]  KtParamMin=[]  KtParamMax=[]  KbOutMin=[]  KbOutMax=[]  KtOutMin=[]  KtOutMax=[]  IntegratorOutMin=[]  IntegratorOutMax=[]  FilterOutMin=[]  FilterOutMax=[]  SumI1OutMin=[]  SumI1OutMax=[]  SumI2OutMin=[]  SumI2OutMax=[]  SumI3OutMin=[]  SumI3OutMax=[]  SumI4OutMin=[]  SumI4OutMax=[]  SumDOutMin=[]  SumDOutMax=[]  DifferentiatorOutMin=[]  DifferentiatorOutMax=[]  FilterDiffOutCoefMin=[]  FilterDiffOutCoefMax=[]  ReciprocalOutMin=[]  ReciprocalOutMax=[]  SumDenOutMin=[]  SumDenOutMax=[]  SumNumOutMin=[]  SumNumOutMax=[]  DivideOutMin=[]  DivideOutMax=[]  UdiffTsProdOutMin=[]  UdiffTsProdOutMax=[]  NTsProdOutMin=[]  NTsProdOutMax=[]  UintegralTsProdOutMin=[]  UintegralTsProdOutMax=[]  UngainTsProdOutMin=[]  UngainTsProdOutMax=[]  ClampingZeroOutDataTypeStr=Inherit: Inherit via back propagation  ClampingZeroOutMin=[]  ClampingZeroOutMax=[]  FilterDenConstantOutDataTypeStr=Inherit: Inherit via back propagation  FilterDenConstantOutMin=[]  FilterDenConstantOutMax=[]  PCopyOutDataTypeStr=Inherit: Inherit via back propagation  PCopyOutMin=[]  PCopyOutMax=[]  NCopyOutDataTypeStr=Inherit: Inherit via back propagation  NCopyOutMin=[]  NCopyOutMax=[]  IntegratorContinuousStateAttributes=''  IntegratorStateMustResolveToSignalObject=off  IntegratorRTWStateStorageClass=Auto  FilterContinuousStateAttributes=''  FilterStateMustResolveToSignalObject=off  FilterRTWStateStorageClass=Auto  ParallelPVariant=InternalParameters  IdealPVariant=Disabled  IVariant=InternalParameters  DVariant=Disabled  IntegratorVariant=Discrete  SatVariant=Disabled  AWVariant=Passthrough  PCopyVariant=Disabled  TRVariant=Disabled  FdbkBlocksVariant=Forward  IdealPFdbkVariant=Disabled  SatFdbkVariant=Disabled  DerivativeFilterVariant=Disabled  NVariant=Disabled  NCopyVariant=Disabled_SignalSpec  FilterICVariant=Disabled  IntegratorICVariant=InternalICs  ExternalResetVariant=Disabled  TRSumVariant=Passthrough  SumFdbkVariant=Disabled  SumVariant=Sum_PI  TsampFilterVariant=InternalTs  TsampNgainVariant=Passthrough  TsampIntegralVariant=Disabled_SignalSpec  ExternalSaturationOutDataTypeStr=Inherit: Same as second input  DerivativeSourceVariant=Disabled  PreIntVariant=InternalPreInt
  Product : Product
  Product1 : Product
  Sum : Sum  Inputs=|+-
  Sum1 : Sum  Inputs=-+|
  Sum2 : Sum  Inputs=+++
  Sum4 : Sum  Inputs=-++
  Terminator : Terminator
  V_abc_c : Outport
  tag scope: y_PI_d_CC=global
  wires:
  Demux2/2 -> Product1/2, Sum1/1
  V_qd/1 -> Demux/1
  Sum1/1 -> PID Controller1/1
  Sum/1 -> PID Controller/1
  Gain/1 -> Product/2, Product1/1
  Demux/2 -> [Vd]
  [Vd] -> Sum4/3
  Mux/1 -> Inverse Park Transformation/1(qd0)
  Constant/1 -> Mux/3
  Demux1/1 -> Sum/1
  Demux2/1 -> Sum/2, Product/1
  theta_g/1 -> Inverse Park Transformation/2(theta)
  Demux/1 -> [Vq]
  PID Controller/1 -> [y_PI_q_CC], Sum2/2
  Product1/1 -> Sum2/3
  [Vq] -> Sum2/1
  Inverse Park Transformation/1(abc) -> V_abc_c/1
  Product/1 -> Sum4/1
  Demux1/2 -> Sum1/2
  w_g/1 -> Gain/1
  I_qd_ref/1 -> Demux1/1
  I_qd_c/1 -> Demux2/1
  Demux2/3 -> Terminator/1
  Sum2/1 -> Delay/1
  Delay/1 -> Mux/1
  Delay1/1 -> Mux/2
  Sum4/1 -> Delay1/1
  PID Controller1/1 -> [y_PI_d_CC], Sum4/2

== system PV_Geno_VSC_GFL_634/PV-Geno with VSC_GFL_at_634     /VSC Control/DC Control ==
  V_dc_ref : Inport
  V_dc : Inport  Port=2
  I_dc : Inport  Port=3
  Gain : Gain
  Gain1 : Gain  Gain=-1
  Gain2 : Gain  Gain=(2/3)*(Vdc/Vp)
  PID Controller : slpidlib/PID Controller  Controller=PI  Form=Parallel  TimeDomain=Discrete-time  UseExternalTs=off  SampleTime=Ts  IntegratorMethod=Forward Euler  FilterMethod=Forward Euler  ControllerParametersSource=internal  P=Kp_DC  I=Ki_DC  UseKiTs=off  D=0  UseExternalDerivativeSource=off  N=100  UseFilter=on  TunerSelectOption=Transfer Function Based (PID Tuner App)  InitialConditionSource=internal  InitialConditionForIntegrator=0  InitialConditionForFilter=0  DifferentiatorICPrevScaledInput=0  ExternalReset=none  TrackingMode=off  Kt=1  LimitOutput=off  SatLimitsSource=internal  UpperSaturationLimit=inf  LowerSaturationLimit=-inf  LinearizeAsGain=on  AntiWindupMode=none  Kb=1  LimitIntegrator=off  UpperIntegratorSaturationLimit=inf  LowerIntegratorSaturationLimit=-inf  POutMin=[]  POutMax=[]  IOutMin=[]  IOutMax=[]  DOutMin=[]  DOutMax=[]  NOutMin=[]  NOutMax=[]  SumOutMin=[]  SumOutMax=[]  SaturationOutMin=[]  SaturationOutMax=[]  PParamMin=[]  PParamMax=[]  IParamMin=[]  IParamMax=[]  DParamMin=[]  DParamMax=[]  NParamMin=[]  NParamMax=[]  KbParamMin=[]  KbParamMax=[]  KtParamMin=[]  KtParamMax=[]  KbOutMin=[]  KbOutMax=[]  KtOutMin=[]  KtOutMax=[]  IntegratorOutMin=[]  IntegratorOutMax=[]  FilterOutMin=[]  FilterOutMax=[]  SumI1OutMin=[]  SumI1OutMax=[]  SumI2OutMin=[]  SumI2OutMax=[]  SumI3OutMin=[]  SumI3OutMax=[]  SumI4OutMin=[]  SumI4OutMax=[]  SumDOutMin=[]  SumDOutMax=[]  DifferentiatorOutMin=[]  DifferentiatorOutMax=[]  FilterDiffOutCoefMin=[]  FilterDiffOutCoefMax=[]  ReciprocalOutMin=[]  ReciprocalOutMax=[]  SumDenOutMin=[]  SumDenOutMax=[]  SumNumOutMin=[]  SumNumOutMax=[]  DivideOutMin=[]  DivideOutMax=[]  UdiffTsProdOutMin=[]  UdiffTsProdOutMax=[]  NTsProdOutMin=[]  NTsProdOutMax=[]  UintegralTsProdOutMin=[]  UintegralTsProdOutMax=[]  UngainTsProdOutMin=[]  UngainTsProdOutMax=[]  ClampingZeroOutDataTypeStr=Inherit: Inherit via back propagation  ClampingZeroOutMin=[]  ClampingZeroOutMax=[]  FilterDenConstantOutDataTypeStr=Inherit: Inherit via back propagation  FilterDenConstantOutMin=[]  FilterDenConstantOutMax=[]  PCopyOutDataTypeStr=Inherit: Inherit via back propagation  PCopyOutMin=[]  PCopyOutMax=[]  NCopyOutDataTypeStr=Inherit: Inherit via back propagation  NCopyOutMin=[]  NCopyOutMax=[]  IntegratorContinuousStateAttributes=''  IntegratorStateMustResolveToSignalObject=off  IntegratorRTWStateStorageClass=Auto  FilterContinuousStateAttributes=''  FilterStateMustResolveToSignalObject=off  FilterRTWStateStorageClass=Auto  ParallelPVariant=InternalParameters  IdealPVariant=Disabled  IVariant=InternalParameters  DVariant=Disabled  IntegratorVariant=Discrete  SatVariant=Disabled  AWVariant=Passthrough  PCopyVariant=Disabled  TRVariant=Disabled  FdbkBlocksVariant=Forward  IdealPFdbkVariant=Disabled  SatFdbkVariant=Disabled  DerivativeFilterVariant=Disabled  NVariant=Disabled  NCopyVariant=Disabled_SignalSpec  FilterICVariant=Disabled  IntegratorICVariant=InternalICs  ExternalResetVariant=Disabled  TRSumVariant=Passthrough  SumFdbkVariant=Disabled  SumVariant=Sum_PI  TsampFilterVariant=InternalTs  TsampNgainVariant=Passthrough  TsampIntegralVariant=Disabled_SignalSpec  ExternalSaturationOutDataTypeStr=Inherit: Same as second input  DerivativeSourceVariant=Disabled  PreIntVariant=InternalPreInt
  Sum : Sum  Inputs=|+-
  Sum1 : Sum  Inputs=|+-
  iq_ref : Outport
  tag scope: y_PI_DC=global
  wires:
  V_dc/1 -> Sum/2
  Sum1/1 -> Gain1/1
  Sum/1 -> PID Controller/1
  I_dc/1 -> Gain/1
  Gain1/1 -> Gain2/1
  Gain2/1 -> iq_ref/1
  Gain/1 -> Sum1/2
  V_dc_ref/1 -> Sum/1
  PID Controller/1 -> [y_PI_DC], Sum1/1

== system PV_Geno_VSC_GFL_634/PV-Geno with VSC_GFL_at_634     /VSC Control/Open-circuit MPPT ==
  T_PV : Inport
  Constant3 : Constant  Value=Tn
  Constant4 : Constant  Value=Voc_n
  Gain : Gain  Gain=KV
  Gain1 : Gain  Gain=KVmp
  Gain2 : Gain  Gain=Ns
  Sum : Sum  Inputs=|++
  Sum1 : Sum  Inputs=|+-
  Vmp : Outport
  wires:
  Gain/1 -> Sum/1
  Constant4/1 -> Sum/2
  Sum/1 -> Gain1/1
  T_PV/1 -> Sum1/1
  Sum1/1 -> Gain/1
  Gain1/1 -> Gain2/1
  Gain2/1 -> Vmp/1
  Constant3/1 -> Sum1/2

== system PV_Geno_VSC_GFL_634/PV-Geno with VSC_GFL_at_634     /VSC Control/PLL ==
  V_abc : Inport
  Constant : Constant  Value=0
  Constant1 : Constant  Value=2*pi*fg
  Demux : Demux  Outputs=3
  Discrete-Time Integrator : DiscreteIntegrator  SampleTime=Ts  ICPrevOutput=DiscIntNeverNeededParam  ICPrevScaledInput=DiscIntNeverNeededParam
  Mux : Mux  Inputs=2
  PID Controller : slpidlib/PID Controller  Controller=PI  Form=Parallel  TimeDomain=Discrete-time  UseExternalTs=off  SampleTime=Ts  IntegratorMethod=Forward Euler  FilterMethod=Forward Euler  ControllerParametersSource=internal  P=Kp_PLL  I=Ki_PLL  UseKiTs=off  D=0  UseExternalDerivativeSource=off  N=100  UseFilter=on  TunerSelectOption=Transfer Function Based (PID Tuner App)  InitialConditionSource=internal  InitialConditionForIntegrator=0  InitialConditionForFilter=0  DifferentiatorICPrevScaledInput=0  ExternalReset=none  TrackingMode=off  Kt=1  LimitOutput=off  SatLimitsSource=internal  UpperSaturationLimit=inf  LowerSaturationLimit=-inf  LinearizeAsGain=on  AntiWindupMode=none  Kb=1  LimitIntegrator=off  UpperIntegratorSaturationLimit=inf  LowerIntegratorSaturationLimit=-inf  POutMin=[]  POutMax=[]  IOutMin=[]  IOutMax=[]  DOutMin=[]  DOutMax=[]  NOutMin=[]  NOutMax=[]  SumOutMin=[]  SumOutMax=[]  SaturationOutMin=[]  SaturationOutMax=[]  PParamMin=[]  PParamMax=[]  IParamMin=[]  IParamMax=[]  DParamMin=[]  DParamMax=[]  NParamMin=[]  NParamMax=[]  KbParamMin=[]  KbParamMax=[]  KtParamMin=[]  KtParamMax=[]  KbOutMin=[]  KbOutMax=[]  KtOutMin=[]  KtOutMax=[]  IntegratorOutMin=[]  IntegratorOutMax=[]  FilterOutMin=[]  FilterOutMax=[]  SumI1OutMin=[]  SumI1OutMax=[]  SumI2OutMin=[]  SumI2OutMax=[]  SumI3OutMin=[]  SumI3OutMax=[]  SumI4OutMin=[]  SumI4OutMax=[]  SumDOutMin=[]  SumDOutMax=[]  DifferentiatorOutMin=[]  DifferentiatorOutMax=[]  FilterDiffOutCoefMin=[]  FilterDiffOutCoefMax=[]  ReciprocalOutMin=[]  ReciprocalOutMax=[]  SumDenOutMin=[]  SumDenOutMax=[]  SumNumOutMin=[]  SumNumOutMax=[]  DivideOutMin=[]  DivideOutMax=[]  UdiffTsProdOutMin=[]  UdiffTsProdOutMax=[]  NTsProdOutMin=[]  NTsProdOutMax=[]  UintegralTsProdOutMin=[]  UintegralTsProdOutMax=[]  UngainTsProdOutMin=[]  UngainTsProdOutMax=[]  ClampingZeroOutDataTypeStr=Inherit: Inherit via back propagation  ClampingZeroOutMin=[]  ClampingZeroOutMax=[]  FilterDenConstantOutDataTypeStr=Inherit: Inherit via back propagation  FilterDenConstantOutMin=[]  FilterDenConstantOutMax=[]  PCopyOutDataTypeStr=Inherit: Inherit via back propagation  PCopyOutMin=[]  PCopyOutMax=[]  NCopyOutDataTypeStr=Inherit: Inherit via back propagation  NCopyOutMin=[]  NCopyOutMax=[]  IntegratorContinuousStateAttributes=''  IntegratorStateMustResolveToSignalObject=off  IntegratorRTWStateStorageClass=Auto  FilterContinuousStateAttributes=''  FilterStateMustResolveToSignalObject=off  FilterRTWStateStorageClass=Auto  ParallelPVariant=InternalParameters  IdealPVariant=Disabled  IVariant=InternalParameters  DVariant=Disabled  IntegratorVariant=Discrete  SatVariant=Disabled  AWVariant=Passthrough  PCopyVariant=Disabled  TRVariant=Disabled  FdbkBlocksVariant=Forward  IdealPFdbkVariant=Disabled  SatFdbkVariant=Disabled  DerivativeFilterVariant=Disabled  NVariant=Disabled  NCopyVariant=Disabled_SignalSpec  FilterICVariant=Disabled  IntegratorICVariant=InternalICs  ExternalResetVariant=Disabled  TRSumVariant=Passthrough  SumFdbkVariant=Disabled  SumVariant=Sum_PI  TsampFilterVariant=InternalTs  TsampNgainVariant=Passthrough  TsampIntegralVariant=Disabled_SignalSpec  ExternalSaturationOutDataTypeStr=Inherit: Same as second input  DerivativeSourceVariant=Disabled  PreIntVariant=InternalPreInt
  Park Transformation : Subsystem
  Sum : Sum  Inputs=|+-
  Sum1 : Sum  Inputs=|++
  Terminator : Terminator
  V_qd : Outport
  w_PLL : Outport  Port=2
  theta_PLL : Outport  Port=3
  tag scope: y_PI_PLL=global
  wires:
  Park Transformation/1(qd0) -> Demux/1
  Demux/3 -> Terminator/1
  PID Controller/1 -> [y_PI_PLL], Sum1/1
  Demux/2 -> Mux/2, Sum/2
  Discrete-Time Integrator/1 -> theta_PLL/1, Park Transformation/2(theta)
  Constant/1 -> Sum/1
  Sum/1 -> PID Controller/1
  Constant1/1 -> Sum1/2
  Sum1/1 -> Discrete-Time Integrator/1, w_PLL/1
  V_abc/1 -> Park Transformation/1(abc)
  Mux/1 -> V_qd/1
  Demux/1 -> Mux/1
